simulink model "VCU_limit_torque"  (R2020a)
settings: Solver=FixedStepDiscrete  StartTime=0.0  StopTime=Parm_cnv_simulink_stopTime  FixedStep=Const_cnv_fundmt_stepSize  RelTol=1e-3  EnableMultiTasking=on
InitFcn:
  | preLoadFun
undefined symbols (not defined in the file or in its folder): IO397
libraries: speedgoatlib_IO691 x8, canmsglib x8, speedgoatlib_fpga x1
Description:
  | - Add preLoadFun.m into Callbacks InitFcn
  | - Combine Sensata and Pirelle sensor inputs into one subsystem
  | - Two enumerators: defEnum_fun_tbm.m && def_vehFun_Enum.m
settings Model: SimulationMode=external  PauseTimes=49.73  NumberOfSteps=20  EnablePacing=on  PacingRate=112  Creator=jianjun.gao  LastModifiedBy=bowen.zheng
settings SolverCC: ConcurrentTasks=on  AlgebraicLoopSolver=LineSearch  AutoInsertRateTranBlk=on
settings DataIOCC: LimitDataPoints=on  SaveFormat=StructureWithTime  ReturnWorkspaceOutputs=off
settings OptimizationCC: BlockReduction=off  DefaultUnderspecifiedDataType=single  OptimizeBlockIOStorage=off  EnhancedBackFolding=on  PassReuseOutputArgsThreshold=0  ExpressionDepthLimit=2147483647  OptimizeBlockOrder=speed  DifferentSizesBufferReuse=on
settings DebuggingCC: UnderspecifiedInitializationDetection=Classic  MergeDetectMultiDrivingBlocksExec=none  SolverPrmCheckMsg=warning  ParameterTunabilityLossMsg=error  FcnCallInpInsideContextMsg=warning  BusObjectLabelMismatch=error  AllowSymbolicDim=off  StateNameClashWarn=warning  SFUnexpectedBacktrackingDiag=warning  SFNoUnconditionalDefaultTransitionDiag=warning  SFExecutionAtInitializationDiag=none  ArithmeticOperatorsInVariantConditions=warning
settings HardwareCC: ProdBitPerPointer=32  ProdBitPerSizeT=32  ProdBitPerPtrDiffT=32  ProdLargestAtomicFloat=None  ProdWordSize=32  ProdLongLongMode=on  ProdHWDeviceType=Generic->32-bit x86 compatible
settings ModelReferenceCC: PropagateSignalLabelsOutOfModel=off
settings SFSimCC: SimUseLocalCustomCode=off  MATLABDynamicMemAlloc=off  CustomCodeUndefinedFunction=UseInterfaceOnly
settings RTWCC: Description=Simulink Real-Time  SystemTargetFile=slrt.tlc  PackageName=addn_compled  TemplateMakefile=slrt_default_tmf  RTWUseLocalCustomCode=off  RTWUseSimCustomCode=on  BuildConfiguration=Faster Runs  CodeExecutionProfiling=on  RTWCompilerOptimization=on
settings CodeAppCC: ForceParamTrailComments=on  MaxIdLength=63  OperatorAnnotations=on
settings SimulinkRealTimeCC: SupportVariableSizeSignals=on  RL32LogTETModifier=off  xPCConcurrentTasks=on
settings ConfigComp: CovMetricSettings=dw  CovHtmlReporting=on  CovSaveCumulativeToWorkspaceVar=on  CovSaveSingleToWorkspaceVar=on  CovExternalEMLEnable=off
settings SimscapeCC: SimscapeNormalizeSystem=off
settings ConfigurationSet: Description=SimMechanics 2G

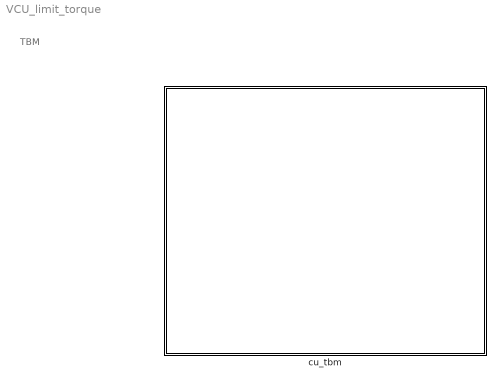
== system VCU_limit_torque ==
  note: TBM
  cu_tbm : Subsystem

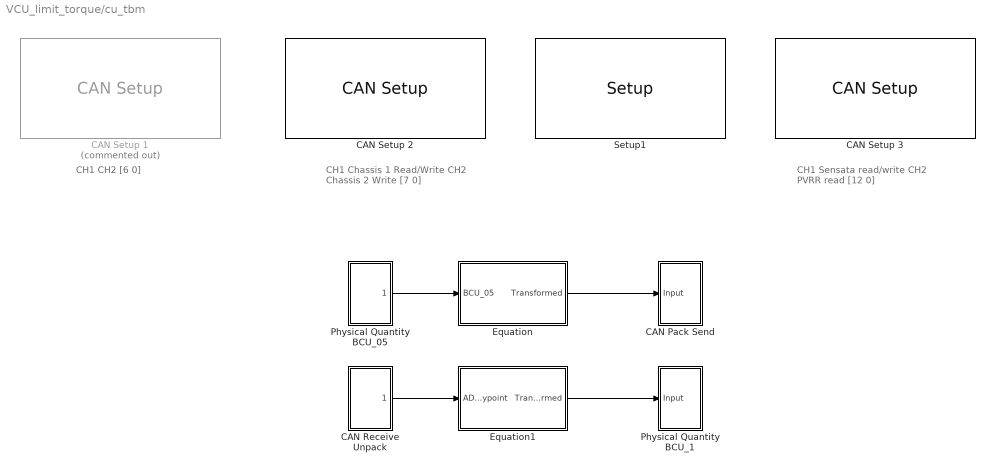
== system VCU_limit_torque/cu_tbm ==
  note: CH1
      | CH2
      | [6 0]
  note: CH1 Chassis 1 Read/Write
      | CH2 Chassis 2 Write
      | [7 0]
  note: CH1 Sensata read/write
      | CH2  PVRR read
      | [12 0]
  CAN Pack Send : Subsystem
  CAN Receive Unpack : Subsystem
  CAN Setup 1 : speedgoatlib_IO691/CAN Setup   Commented=on  moduletype=IO691  id=1  pciSlot=[6 0]  chn1=CAN (HS)  chn2=CAN (HS)  chn3=Disabled  chn4=Disabled  initStruct=[]  termStruct=[]  ArbitrationbdrChn1=500 kBaud  ArbitrationManbdrChn1=[2,16,63,16]  FdbdrChn1=5.0 MBaud  FdManbdrChn1=[2,2,5,2]  ArbitrationbdrChn2=500 kBaud  ArbitrationManbdrChn2=[2,16,63,16]  FdbdrChn2=5.0 MBaud  FdManbdrChn2=[2,2,5,2]  ArbitrationbdrChn3=1.0 MBaud  ArbitrationManbdrChn3=[2,8,31,8]  FdbdrChn3=5.0 MBaud  FdManbdrChn3=[2,2,5,2]  ArbitrationbdrChn4=1.0 MBaud  ArbitrationManbdrChn4=[2,8,31,8]  FdbdrChn4=5.0 MBaud  FdManbdrChn4=[2,2,5,2]  moduleInitValues=[691 1 6 0]
      settings: SourceProductName=Simulink Real-Time: Speedgoat I/O Blockset
  CAN Setup 2 : speedgoatlib_IO691/CAN Setup   moduletype=IO691  id=2  pciSlot=[7 0]  chn1=CAN (HS)  chn2=CAN (HS)  chn3=Disabled  chn4=Disabled  initStruct=[]  termStruct=[]  ArbitrationbdrChn1=500 kBaud  ArbitrationManbdrChn1=[2,16,63,16]  FdbdrChn1=5.0 MBaud  FdManbdrChn1=[2,2,5,2]  ArbitrationbdrChn2=500 kBaud  ArbitrationManbdrChn2=[2,16,63,16]  FdbdrChn2=5.0 MBaud  FdManbdrChn2=[2,2,5,2]  ArbitrationbdrChn3=1.0 MBaud  ArbitrationManbdrChn3=[2,8,31,8]  FdbdrChn3=5.0 MBaud  FdManbdrChn3=[2,2,5,2]  ArbitrationbdrChn4=1.0 MBaud  ArbitrationManbdrChn4=[2,8,31,8]  FdbdrChn4=5.0 MBaud  FdManbdrChn4=[2,2,5,2]  moduleInitValues=[691 2 7 0]
      settings: SourceProductName=Simulink Real-Time: Speedgoat I/O Blockset
  CAN Setup 3 : speedgoatlib_IO691/CAN Setup   moduletype=IO691  id=4  pciSlot=[12 0]  chn1=CAN (HS)  chn2=CAN (HS)  chn3=Disabled  chn4=Disabled  initStruct=[]  termStruct=[]  ArbitrationbdrChn1=500 kBaud  ArbitrationManbdrChn1=[2,16,63,16]  FdbdrChn1=5.0 MBaud  FdManbdrChn1=[2,2,5,2]  ArbitrationbdrChn2=1.0 MBaud  ArbitrationManbdrChn2=[2,8,31,8]  FdbdrChn2=5.0 MBaud  FdManbdrChn2=[2,2,5,2]  ArbitrationbdrChn3=1.0 MBaud  ArbitrationManbdrChn3=[2,8,31,8]  FdbdrChn3=5.0 MBaud  FdManbdrChn3=[2,2,5,2]  ArbitrationbdrChn4=1.0 MBaud  ArbitrationManbdrChn4=[2,8,31,8]  FdbdrChn4=5.0 MBaud  FdManbdrChn4=[2,2,5,2]  moduleInitValues=[691 4 12 0]
      settings: SourceProductName=Simulink Real-Time: Speedgoat I/O Blockset
  Equation : Subsystem
  Equation1 : Subsystem
  Physical Quantity BCU_05 : Subsystem
  Physical Quantity BCU_1 : Subsystem
  Setup1 : speedgoatlib_fpga/Setup/Setup  board=IO397-50k  id=3  device_id=1  frontIO=None  rearIO=None  bitstreamFile=speedgoat_IO397_50k_all_io.mat  rev=2.1  timestamp_string=06/12/19 11:07:30  fpgaFreq=75 MHz  fpgaTick=13.33 ns  ProgSpiFlash=off  ProgBPIFlash=off  pciSlot=-1  PullRPort0=pull-up 3.3V  VioPort0=3.3V  PullRPort1=pull-up 3.3V  VioPort1=3.3V  PullRPort2=pull-up 3.3V  VioPort2=3.3V  PullRPort3=pull-up 3.3V  VioPort3=3.3V  PullRPort4=pull-up 3.3V  VioPort4=3.3V  PullRPort5=pull-up 3.3V  VioPort5=3.3V  PullRPort6=pull-up 3.3V  VioPort6=3.3V  PullRPort15=pull-up 3.3V  PullRPort31=pull-up 3.3V  PullRPort47=pull-up 3.3V  PullRPort63=pull-up 3.3V
      settings: SourceProductName=Simulink Real-Time: Speedgoat Library
  wires:
  Physical Quantity BCU_05/1(BCU_05) -> Equation/1(BCU_05)
  Equation/1(Transformed) -> CAN Pack Send/1(Input)
  CAN Receive Unpack/1(Output) -> Equation1/1(ADC_Waypoint)
  Equation1/1(Transformed) -> Physical Quantity BCU_1/1(Input)

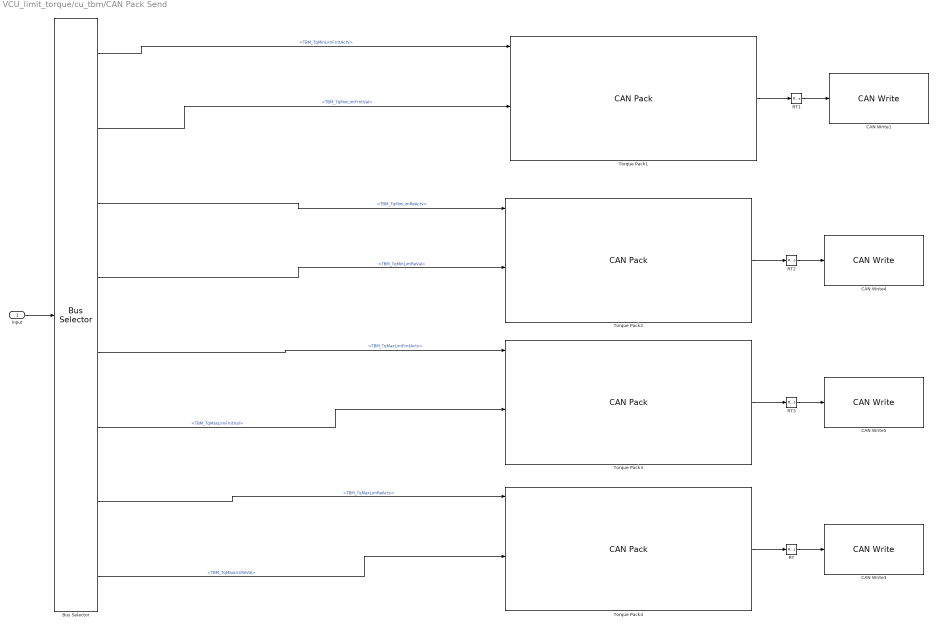
== system VCU_limit_torque/cu_tbm/CAN Pack Send ==
  Input : Inport
  Bus Selector : BusSelector  OutputSignals=TBM_TqMinLimFrntActv,TBM_TqMinLimFrntVal,TBM_TqMinLimReActv,TBM_TqMinLimReVal,TBM_TqMaxLimFrntActv,TBM_TqMaxLimFrntVal,TBM_TqMaxLimReActv,TBM_TqMaxLimReVal
  CAN Write{1,3..5} (4 alike) : speedgoatlib_IO691/CAN Write  id=2  ts=0.02  channel=1  messageType=CAN  enableStatusPort=off  canType=CAN (HS)  initValues=[691 2 0.02 0 1 1 0]
      settings: SourceProductName=Simulink Real-Time: Speedgoat I/O Blockset
  RT{,1..3} (4 alike) : RateTransition  OutPortSampleTime=0.02
  Torque Pack1 : canmsglib/CAN Pack  CANdbFile=.\support\dbc\NIO_NT2_Chassis2_CAN_Official_Release_V_1_1_DA_02.dbc  MsgList=ADC1_WayPoint01  MsgName=ADC1_WayPoint01  MsgIDType=Standard (11-bit identifier)  MsgIdentifier=214  MsgLength=8  Remote=off  ApplyMinMax=off  BusOutput=off  SignalInfo={'LD_Confidence_1','24','4','BE','unsigned','Standard','0','0.1','0','0','1.5';'LD_First_End_1','51','7','BE','unsigned','Standard','0','1','0','0','127';'LD_First_Start_1','16','8','BE','unsigned','Standard','0','0.1','0','0','25.5';'LD_First_Type_1','28','4','BE','unsigned','Standard','0','1','0','0','15';'LD_Line_First_C0_1','56','11','BE','unsigned','Standard','0','0.01','-10.24','-10.24','10.23';'LD_Line_First_C1_1','43','13','BE','unsigned','Standard','0','0.0001','-0.4096','-0.4096','0.4095';'LD_Line_First_C2_1','0','8','BE','unsigned','Standard','0','0.0001','-0.0128','-0.0128','0.0127';'LD_Line_First_C3_1','8','8','BE','unsigned','Standard','0','1e-06','-0.000128','-0.000128','0.000127'}
      settings: SourceProductBaseCode=ME,VN  DataFormat=CANdb specified signals
  Torque Pack2 : canmsglib/CAN Pack  CANdbFile=.\support\dbc\NIO_NT2_Chassis2_CAN_Official_Release_V_1_1_DA_02.dbc  MsgList=ADC1_WayPoint02  MsgName=ADC1_WayPoint02  MsgIDType=Standard (11-bit identifier)  MsgIdentifier=215  MsgLength=8  Remote=off  ApplyMinMax=off  BusOutput=off  SignalInfo={'LD_Confidence_2','24','4','BE','unsigned','Standard','0','0.1','0','0','1.5';'LD_First_End_2','51','7','BE','unsigned','Standard','0','1','0','0','127';'LD_First_Start_2','16','8','BE','unsigned','Standard','0','0.1','0','0','25.5';'LD_First_Type_2','28','4','BE','unsigned','Standard','0','1','0','0','15';'LD_Line_First_C0_2','56','11','BE','unsigned','Standard','0','0.01','-10.24','-10.24','10.23';'LD_Line_First_C1_2','43','13','BE','unsigned','Standard','0','0.0001','-0.4096','-0.4096','0.4095';'LD_Line_First_C2_2','0','8','BE','unsigned','Standard','0','0.0001','-0.0128','-0.0128','0.0127';'LD_Line_First_C3_2','8','8','BE','unsigned','Standard','0','1e-06','-0.000128','-0.000128','0.000127'}
      settings: SourceProductBaseCode=ME,VN  DataFormat=CANdb specified signals
  Torque Pack3 : canmsglib/CAN Pack  CANdbFile=.\support\dbc\NIO_NT2_Chassis2_CAN_Official_Release_V_1_1_DA_02.dbc  MsgList=ADC1_WayPoint03  MsgName=ADC1_WayPoint03  MsgIDType=Standard (11-bit identifier)  MsgIdentifier=216  MsgLength=8  Remote=off  ApplyMinMax=off  BusOutput=off  SignalInfo={'LD_Confidence_3','24','4','BE','unsigned','Standard','0','0.1','0','0','1.5';'LD_First_End_3','51','7','BE','unsigned','Standard','0','1','0','0','127';'LD_First_Start_3','16','8','BE','unsigned','Standard','0','0.1','0','0','25.5';'LD_First_Type_3','28','4','BE','unsigned','Standard','0','1','0','0','15';'LD_Line_First_C0_3','56','11','BE','unsigned','Standard','0','0.01','-10.24','-10.24','10.23';'LD_Line_First_C1_3','43','13','BE','unsigned','Standard','0','0.0001','-0.4096','-0.4096','0.4095';'LD_Line_First_C2_3','0','8','BE','unsigned','Standard','0','0.0001','-0.0128','-0.0128','0.0127';'LD_Line_First_C3_3','8','8','BE','unsigned','Standard','0','1e-06','-0.000128','-0.000128','0.000127'}
      settings: SourceProductBaseCode=ME,VN  DataFormat=CANdb specified signals
  Torque Pack4 : canmsglib/CAN Pack  CANdbFile=.\support\dbc\NIO_NT2_Chassis2_CAN_Official_Release_V_1_1_DA_02.dbc  MsgList=ADC1_WayPoint04  MsgName=ADC1_WayPoint04  MsgIDType=Standard (11-bit identifier)  MsgIdentifier=217  MsgLength=8  Remote=off  ApplyMinMax=off  BusOutput=off  SignalInfo={'LD_Confidence_4','24','4','BE','unsigned','Standard','0','0.1','0','0','1.5';'LD_First_End_4','51','7','BE','unsigned','Standard','0','1','0','0','127';'LD_First_Start_4','16','8','BE','unsigned','Standard','0','0.1','0','0','25.5';'LD_First_Type_4','28','4','BE','unsigned','Standard','0','1','0','0','15';'LD_Line_First_C0_4','56','11','BE','unsigned','Standard','0','0.01','-10.24','-10.24','10.23';'LD_Line_First_C1_4','43','13','BE','unsigned','Standard','0','0.0001','-0.4096','-0.4096','0.4095';'LD_Line_First_C2_4','0','8','BE','unsigned','Standard','0','0.0001','-0.0128','-0.0128','0.0127';'LD_Line_First_C3_4','8','8','BE','unsigned','Standard','0','1e-06','-0.000128','-0.000128','0.000127'}
      settings: SourceProductBaseCode=ME,VN  DataFormat=CANdb specified signals
  wires:
  RT/1 -> CAN Write3/1
  RT3/1 -> CAN Write5/1
  Torque Pack3/1 -> RT3/1
  Torque Pack4/1 -> RT/1
  Torque Pack2/1 -> RT2/1
  RT2/1 -> CAN Write4/1
  Input/1 -> Bus Selector/1
  Bus Selector/1 -> Torque Pack1/1  "<TBM_TqMinLimFrntActv>"
  RT1/1 -> CAN Write1/1
  Torque Pack1/1 -> RT1/1
  Bus Selector/2 -> Torque Pack1/5  "<TBM_TqMinLimFrntVal>"
  Bus Selector/3 -> Torque Pack2/1  "<TBM_TqMinLimReActv>"
  Bus Selector/4 -> Torque Pack2/5  "<TBM_TqMinLimReVal>"
  Bus Selector/5 -> Torque Pack3/1  "<TBM_TqMaxLimFrntActv>"
  Bus Selector/6 -> Torque Pack3/5  "<TBM_TqMaxLimFrntVal>"
  Bus Selector/7 -> Torque Pack4/1  "<TBM_TqMaxLimReActv>"
  Bus Selector/8 -> Torque Pack4/5  "<TBM_TqMaxLimReVal>"

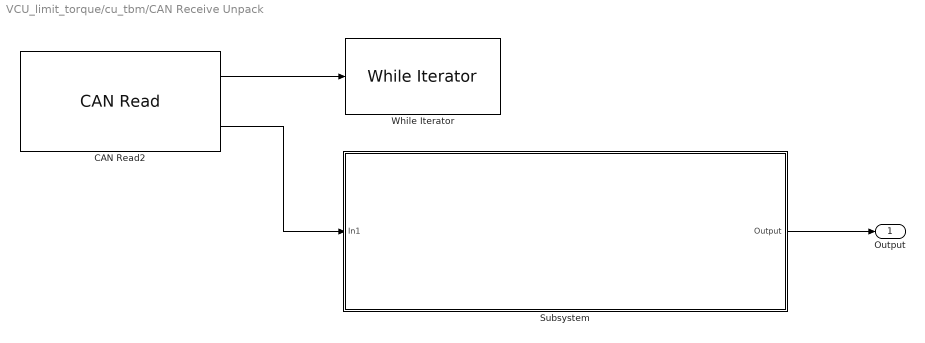
== system VCU_limit_torque/cu_tbm/CAN Receive Unpack ==
  CAN Read2 : speedgoatlib_IO691/CAN Read  id=2  ts=-1  channel=1  messageType=CAN  canType=CAN (HS)  initValues=[691 2 -1 0 1 1]
      settings: SourceProductName=Simulink Real-Time: Speedgoat I/O Blockset
  Subsystem : Subsystem
  While Iterator : WhileIterator  MaxIters=-1  WhileBlockType=do-while
  Output : Outport
  wires:
  CAN Read2/2 -> Subsystem/1(In1)
  CAN Read2/1 -> While Iterator/1
  Subsystem/1(Output) -> Output/1

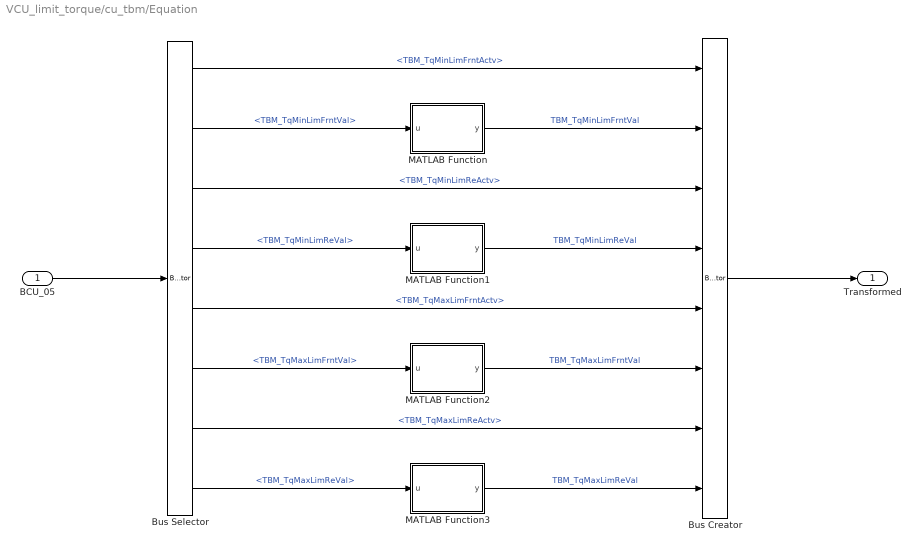
== system VCU_limit_torque/cu_tbm/Equation ==
  BCU_05 : Inport
  Bus Creator : BusCreator  Inputs=8
  Bus Selector : BusSelector  OutputSignals=TBM_TqMinLimFrntActv,TBM_TqMinLimFrntVal,TBM_TqMinLimReActv,TBM_TqMinLimReVal,TBM_TqMaxLimFrntActv,TBM_TqMaxLimFrntVal,TBM_TqMaxLimReActv,TBM_TqMaxLimReVal
  MATLAB Function : MATLAB Function  TreatAsAtomicUnit=on
  MATLAB Function1 : MATLAB Function  TreatAsAtomicUnit=on
  MATLAB Function2 : MATLAB Function  TreatAsAtomicUnit=on
  MATLAB Function3 : MATLAB Function  TreatAsAtomicUnit=on
  Transformed : Outport
  wires:
  BCU_05/1 -> Bus Selector/1
  Bus Creator/1 -> Transformed/1
  Bus Selector/1 -> Bus Creator/1  "<TBM_TqMinLimFrntActv>"
  Bus Selector/3 -> Bus Creator/3  "<TBM_TqMinLimReActv>"
  Bus Selector/5 -> Bus Creator/5  "<TBM_TqMaxLimFrntActv>"
  Bus Selector/7 -> Bus Creator/7  "<TBM_TqMaxLimReActv>"
  Bus Selector/2 -> MATLAB Function/1(u)  "<TBM_TqMinLimFrntVal>"
  MATLAB Function/1(y) -> Bus Creator/2  "TBM_TqMinLimFrntVal"
  Bus Selector/8 -> MATLAB Function3/1(u)  "<TBM_TqMaxLimReVal>"
  Bus Selector/6 -> MATLAB Function2/1(u)  "<TBM_TqMaxLimFrntVal>"
  Bus Selector/4 -> MATLAB Function1/1(u)  "<TBM_TqMinLimReVal>"
  MATLAB Function1/1(y) -> Bus Creator/4  "TBM_TqMinLimReVal"
  MATLAB Function2/1(y) -> Bus Creator/6  "TBM_TqMaxLimFrntVal"
  MATLAB Function3/1(y) -> Bus Creator/8  "TBM_TqMaxLimReVal"

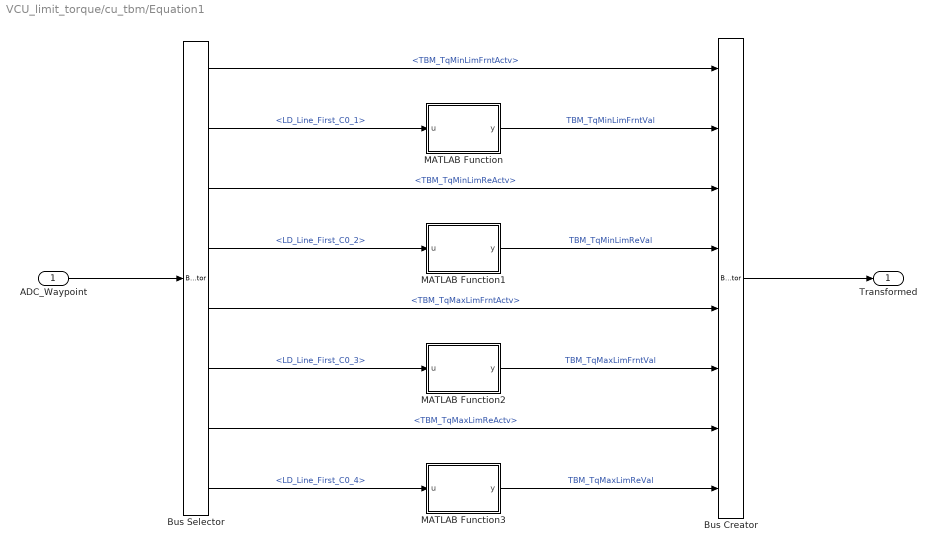
== system VCU_limit_torque/cu_tbm/Equation1 ==
  ADC_Waypoint : Inport
  Bus Creator : BusCreator  Inputs=8
  Bus Selector : BusSelector  OutputSignals=TBM_TqMinLimFrntActv,LD_Line_First_C0_1,TBM_TqMinLimReActv,LD_Line_First_C0_2,TBM_TqMaxLimFrntActv,LD_Line_First_C0_3,TBM_TqMaxLimReActv,LD_Line_First_C0_4
  MATLAB Function : MATLAB Function  TreatAsAtomicUnit=on
  MATLAB Function1 : MATLAB Function  TreatAsAtomicUnit=on
  MATLAB Function2 : MATLAB Function  TreatAsAtomicUnit=on
  MATLAB Function3 : MATLAB Function  TreatAsAtomicUnit=on
  Transformed : Outport
  wires:
  ADC_Waypoint/1 -> Bus Selector/1
  Bus Creator/1 -> Transformed/1
  Bus Selector/1 -> Bus Creator/1  "<TBM_TqMinLimFrntActv>"
  Bus Selector/3 -> Bus Creator/3  "<TBM_TqMinLimReActv>"
  Bus Selector/5 -> Bus Creator/5  "<TBM_TqMaxLimFrntActv>"
  Bus Selector/7 -> Bus Creator/7  "<TBM_TqMaxLimReActv>"
  Bus Selector/2 -> MATLAB Function/1(u)  "<LD_Line_First_C0_1>"
  MATLAB Function/1(y) -> Bus Creator/2  "TBM_TqMinLimFrntVal"
  Bus Selector/8 -> MATLAB Function3/1(u)  "<LD_Line_First_C0_4>"
  Bus Selector/6 -> MATLAB Function2/1(u)  "<LD_Line_First_C0_3>"
  Bus Selector/4 -> MATLAB Function1/1(u)  "<LD_Line_First_C0_2>"
  MATLAB Function1/1(y) -> Bus Creator/4  "TBM_TqMinLimReVal"
  MATLAB Function2/1(y) -> Bus Creator/6  "TBM_TqMaxLimFrntVal"
  MATLAB Function3/1(y) -> Bus Creator/8  "TBM_TqMaxLimReVal"

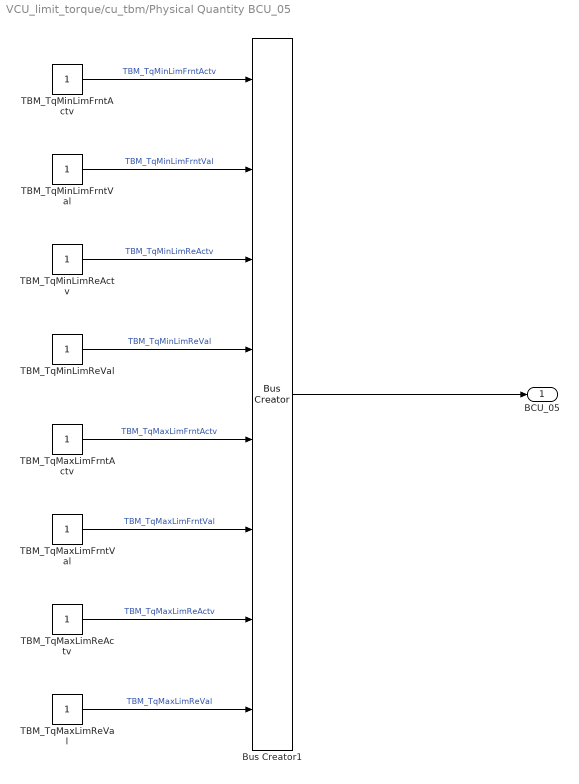
== system VCU_limit_torque/cu_tbm/Physical Quantity BCU_05 ==
  Bus Creator1 : BusCreator  Inputs=8
  TBM_TqMaxLimFrntActv : Constant  OutDataTypeStr=single
  TBM_TqMaxLimFrntVal : Constant  OutDataTypeStr=single
  TBM_TqMaxLimReActv : Constant  OutDataTypeStr=single
  TBM_TqMaxLimReVal : Constant  OutDataTypeStr=single
  TBM_TqMinLimFrntActv : Constant  OutDataTypeStr=single
  TBM_TqMinLimFrntVal : Constant  OutDataTypeStr=single
  TBM_TqMinLimReActv : Constant  OutDataTypeStr=single
  TBM_TqMinLimReVal : Constant  OutDataTypeStr=single
  BCU_05 : Outport  OutDataTypeStr=single  PortDimensions=8
  wires:
  TBM_TqMaxLimReVal/1 -> Bus Creator1/8  "TBM_TqMaxLimReVal"
  Bus Creator1/1 -> BCU_05/1
  TBM_TqMinLimFrntVal/1 -> Bus Creator1/2  "TBM_TqMinLimFrntVal"
  TBM_TqMinLimReVal/1 -> Bus Creator1/4  "TBM_TqMinLimReVal"
  TBM_TqMinLimReActv/1 -> Bus Creator1/3  "TBM_TqMinLimReActv"
  TBM_TqMaxLimFrntActv/1 -> Bus Creator1/5  "TBM_TqMaxLimFrntActv"
  TBM_TqMaxLimReActv/1 -> Bus Creator1/7  "TBM_TqMaxLimReActv"
  TBM_TqMinLimFrntActv/1 -> Bus Creator1/1  "TBM_TqMinLimFrntActv"
  TBM_TqMaxLimFrntVal/1 -> Bus Creator1/6  "TBM_TqMaxLimFrntVal"

== system VCU_limit_torque/cu_tbm/Physical Quantity BCU_1 ==
  Input : Inport
  Bus Selector : BusSelector  OutputSignals=TBM_TqMinLimFrntActv,TBM_TqMinLimFrntVal,TBM_TqMinLimReActv,TBM_TqMinLimReVal,TBM_TqMaxLimFrntActv,TBM_TqMaxLimFrntVal,TBM_TqMaxLimReActv,TBM_TqMaxLimReVal
  wires:
  Bus Selector/8 -> ?  "<TBM_TqMaxLimReVal>"
  Bus Selector/2 -> ?  "<TBM_TqMinLimFrntVal>"
  Bus Selector/4 -> ?  "<TBM_TqMinLimReVal>"
  Bus Selector/3 -> ?  "<TBM_TqMinLimReActv>"
  Bus Selector/5 -> ?  "<TBM_TqMaxLimFrntActv>"
  Bus Selector/7 -> ?  "<TBM_TqMaxLimReActv>"
  Bus Selector/1 -> ?  "<TBM_TqMinLimFrntActv>"
  Bus Selector/6 -> ?  "<TBM_TqMaxLimFrntVal>"
  Input/1 -> Bus Selector/1

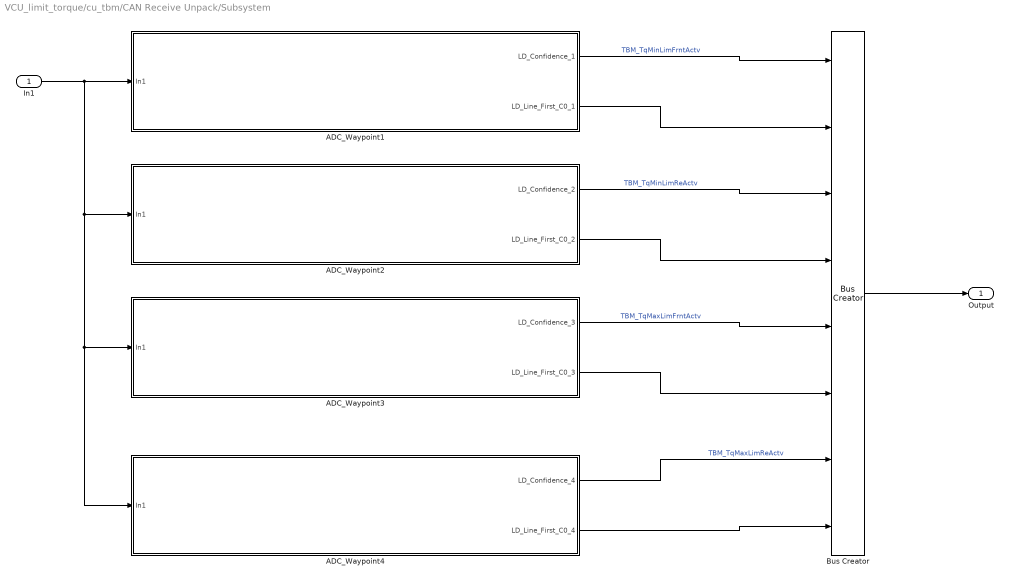
== system VCU_limit_torque/cu_tbm/CAN Receive Unpack/Subsystem ==
  In1 : Inport
  ADC_Waypoint1 : Subsystem
  ADC_Waypoint2 : Subsystem
  ADC_Waypoint3 : Subsystem
  ADC_Waypoint4 : Subsystem
  Bus Creator : BusCreator  Inputs=8
  Output : Outport
  wires:
  In1/1 -> ADC_Waypoint4/1(In1), ADC_Waypoint3/1(In1), ADC_Waypoint2/1(In1), ADC_Waypoint1/1(In1)
  ADC_Waypoint1/1(LD_Confidence_1) -> Bus Creator/1  "TBM_TqMinLimFrntActv"
  ADC_Waypoint1/2(LD_Line_First_C0_1) -> Bus Creator/2
  ADC_Waypoint2/1(LD_Confidence_2) -> Bus Creator/3  "TBM_TqMinLimReActv"
  ADC_Waypoint2/2(LD_Line_First_C0_2) -> Bus Creator/4
  ADC_Waypoint3/1(LD_Confidence_3) -> Bus Creator/5  "TBM_TqMaxLimFrntActv"
  ADC_Waypoint3/2(LD_Line_First_C0_3) -> Bus Creator/6
  ADC_Waypoint4/1(LD_Confidence_4) -> Bus Creator/7  "TBM_TqMaxLimReActv"
  ADC_Waypoint4/2(LD_Line_First_C0_4) -> Bus Creator/8
  Bus Creator/1 -> Output/1

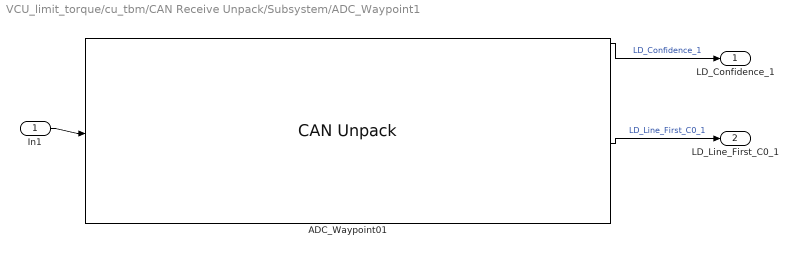
== system VCU_limit_torque/cu_tbm/CAN Receive Unpack/Subsystem/ADC_Waypoint1 ==
  In1 : Inport
  ADC_Waypoint01 : canmsglib/CAN Unpack  CANdbFile=C:\Users\bowen.zheng\Desktop\spdGoat_prj_20230605\spdGoat_prj_20230605\support\dbc\NIO_NT2_Chassis2_CAN_Official_Release_V_1_1_DA_02.dbc  MsgList=ADC1_WayPoint01  MsgName=ADC1_WayPoint01  MsgIDType=Standard (11-bit identifier)  MsgIdentifier=214  MsgLength=8  SignalInfo={'LD_Confidence_1','24','4','BE','unsigned','Standard','0','0.1','0','0','1.5';'LD_First_End_1','51','7','BE','unsigned','Standard','0','1','0','0','127';'LD_First_Start_1','16','8','BE','unsigned','Standard','0','0.1','0','0','25.5';'LD_First_Type_1','28','4','BE','unsigned','Standard','0','1','0','0','15';'LD_Line_First_C0_1','56','11','BE','unsigned','Standard','0','0.01','-10.24','-10.24','10.23';'LD_Line_First_C1_1','43','13','BE','unsigned','Standard','0','0.0001','-0.4096','-0.4096','0.4095';'LD_Line_First_C2_1','0','8','BE','unsigned','Standard','0','0.0001','-0.0128','-0.0128','0.0127';'LD_Line_First_C3_1','8','8','BE','unsigned','Standard','0','1e-06','-0.000128','-0.000128','0.000127'}  IDPort=off  TimestampPort=off  ErrorPort=off  RemotePort=off  LengthPort=off  StatusPort=off  ApplyMinMax=off
      settings: SourceProductBaseCode=ME,VN  DataFormat=CANdb specified signals
  LD_Confidence_1 : Outport
  LD_Line_First_C0_1 : Outport  Port=2
  wires:
  In1/1 -> ADC_Waypoint01/1
  ADC_Waypoint01/1 -> LD_Confidence_1/1  "LD_Confidence_1"
  ADC_Waypoint01/5 -> LD_Line_First_C0_1/1  "LD_Line_First_C0_1"

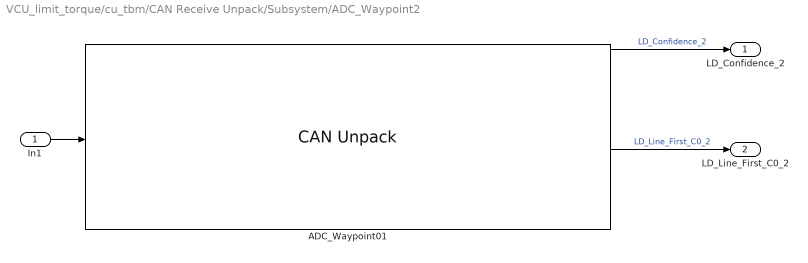
== system VCU_limit_torque/cu_tbm/CAN Receive Unpack/Subsystem/ADC_Waypoint2 ==
  In1 : Inport
  ADC_Waypoint01 : canmsglib/CAN Unpack  CANdbFile=C:\Users\bowen.zheng\Desktop\spdGoat_prj_20230605\spdGoat_prj_20230605\support\dbc\NIO_NT2_Chassis2_CAN_Official_Release_V_1_1_DA_02.dbc  MsgList=ADC1_WayPoint02  MsgName=ADC1_WayPoint02  MsgIDType=Standard (11-bit identifier)  MsgIdentifier=215  MsgLength=8  SignalInfo={'LD_Confidence_2','24','4','BE','unsigned','Standard','0','0.1','0','0','1.5';'LD_First_End_2','51','7','BE','unsigned','Standard','0','1','0','0','127';'LD_First_Start_2','16','8','BE','unsigned','Standard','0','0.1','0','0','25.5';'LD_First_Type_2','28','4','BE','unsigned','Standard','0','1','0','0','15';'LD_Line_First_C0_2','56','11','BE','unsigned','Standard','0','0.01','-10.24','-10.24','10.23';'LD_Line_First_C1_2','43','13','BE','unsigned','Standard','0','0.0001','-0.4096','-0.4096','0.4095';'LD_Line_First_C2_2','0','8','BE','unsigned','Standard','0','0.0001','-0.0128','-0.0128','0.0127';'LD_Line_First_C3_2','8','8','BE','unsigned','Standard','0','1e-06','-0.000128','-0.000128','0.000127'}  IDPort=off  TimestampPort=off  ErrorPort=off  RemotePort=off  LengthPort=off  StatusPort=off  ApplyMinMax=off
      settings: SourceProductBaseCode=ME,VN  DataFormat=CANdb specified signals
  LD_Confidence_2 : Outport
  LD_Line_First_C0_2 : Outport  Port=2
  wires:
  In1/1 -> ADC_Waypoint01/1
  ADC_Waypoint01/1 -> LD_Confidence_2/1  "LD_Confidence_2"
  ADC_Waypoint01/5 -> LD_Line_First_C0_2/1  "LD_Line_First_C0_2"

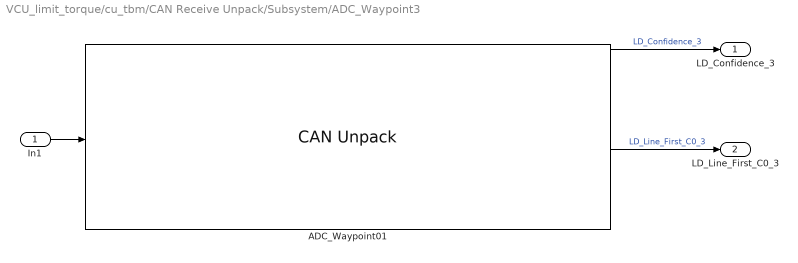
== system VCU_limit_torque/cu_tbm/CAN Receive Unpack/Subsystem/ADC_Waypoint3 ==
  In1 : Inport
  ADC_Waypoint01 : canmsglib/CAN Unpack  CANdbFile=C:\Users\bowen.zheng\Desktop\spdGoat_prj_20230605\spdGoat_prj_20230605\support\dbc\NIO_NT2_Chassis2_CAN_Official_Release_V_1_1_DA_02.dbc  MsgList=ADC1_WayPoint03  MsgName=ADC1_WayPoint03  MsgIDType=Standard (11-bit identifier)  MsgIdentifier=216  MsgLength=8  SignalInfo={'LD_Confidence_3','24','4','BE','unsigned','Standard','0','0.1','0','0','1.5';'LD_First_End_3','51','7','BE','unsigned','Standard','0','1','0','0','127';'LD_First_Start_3','16','8','BE','unsigned','Standard','0','0.1','0','0','25.5';'LD_First_Type_3','28','4','BE','unsigned','Standard','0','1','0','0','15';'LD_Line_First_C0_3','56','11','BE','unsigned','Standard','0','0.01','-10.24','-10.24','10.23';'LD_Line_First_C1_3','43','13','BE','unsigned','Standard','0','0.0001','-0.4096','-0.4096','0.4095';'LD_Line_First_C2_3','0','8','BE','unsigned','Standard','0','0.0001','-0.0128','-0.0128','0.0127';'LD_Line_First_C3_3','8','8','BE','unsigned','Standard','0','1e-06','-0.000128','-0.000128','0.000127'}  IDPort=off  TimestampPort=off  ErrorPort=off  RemotePort=off  LengthPort=off  StatusPort=off  ApplyMinMax=off
      settings: SourceProductBaseCode=ME,VN  DataFormat=CANdb specified signals
  LD_Confidence_3 : Outport
  LD_Line_First_C0_3 : Outport  Port=2
  wires:
  In1/1 -> ADC_Waypoint01/1
  ADC_Waypoint01/1 -> LD_Confidence_3/1  "LD_Confidence_3"
  ADC_Waypoint01/5 -> LD_Line_First_C0_3/1  "LD_Line_First_C0_3"

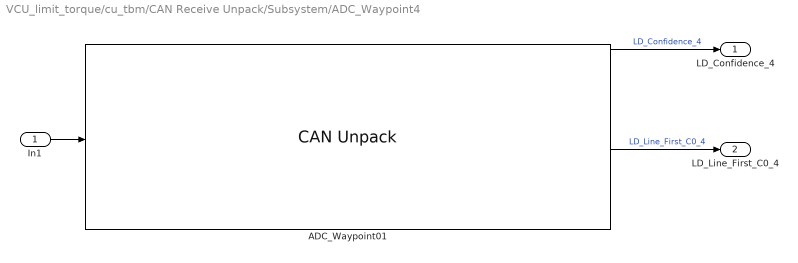
== system VCU_limit_torque/cu_tbm/CAN Receive Unpack/Subsystem/ADC_Waypoint4 ==
  In1 : Inport
  ADC_Waypoint01 : canmsglib/CAN Unpack  CANdbFile=C:\Users\bowen.zheng\Desktop\spdGoat_prj_20230605\spdGoat_prj_20230605\support\dbc\NIO_NT2_Chassis2_CAN_Official_Release_V_1_1_DA_02.dbc  MsgList=ADC1_WayPoint04  MsgName=ADC1_WayPoint04  MsgIDType=Standard (11-bit identifier)  MsgIdentifier=217  MsgLength=8  SignalInfo={'LD_Confidence_4','24','4','BE','unsigned','Standard','0','0.1','0','0','1.5';'LD_First_End_4','51','7','BE','unsigned','Standard','0','1','0','0','127';'LD_First_Start_4','16','8','BE','unsigned','Standard','0','0.1','0','0','25.5';'LD_First_Type_4','28','4','BE','unsigned','Standard','0','1','0','0','15';'LD_Line_First_C0_4','56','11','BE','unsigned','Standard','0','0.01','-10.24','-10.24','10.23';'LD_Line_First_C1_4','43','13','BE','unsigned','Standard','0','0.0001','-0.4096','-0.4096','0.4095';'LD_Line_First_C2_4','0','8','BE','unsigned','Standard','0','0.0001','-0.0128','-0.0128','0.0127';'LD_Line_First_C3_4','8','8','BE','unsigned','Standard','0','1e-06','-0.000128','-0.000128','0.000127'}  IDPort=off  TimestampPort=off  ErrorPort=off  RemotePort=off  LengthPort=off  StatusPort=off  ApplyMinMax=off
      settings: SourceProductBaseCode=ME,VN  DataFormat=CANdb specified signals
  LD_Confidence_4 : Outport
  LD_Line_First_C0_4 : Outport  Port=2
  wires:
  In1/1 -> ADC_Waypoint01/1
  ADC_Waypoint01/1 -> LD_Confidence_4/1  "LD_Confidence_4"
  ADC_Waypoint01/5 -> LD_Line_First_C0_4/1  "LD_Line_First_C0_4"

== matlab function VCU_limit_torque/cu_tbm/Equation/MATLAB Function1 ==
  data: u input; y output
function y = fcn(u)

 y = 0.01 * u - 6.04;

== matlab function VCU_limit_torque/cu_tbm/Equation/MATLAB Function2 ==
  data: u input; y output
function y = fcn(u)

 y = 0.01 * u - 6.04;

== matlab function VCU_limit_torque/cu_tbm/Equation/MATLAB Function3 ==
  data: u input; y output
function y = fcn(u)

 y = 0.01 * u - 6.04;

== matlab function VCU_limit_torque/cu_tbm/Equation1/MATLAB Function ==
  data: u input; y output
function y = fcn(u)

 y = (u + 6.04) / 0.01;

== matlab function VCU_limit_torque/cu_tbm/Equation1/MATLAB Function1 ==
  data: u input; y output
function y = fcn(u)

 y = (u + 6.04) / 0.01;

== matlab function VCU_limit_torque/cu_tbm/Equation1/MATLAB Function2 ==
  data: u input; y output
function y = fcn(u)

 y = (u + 6.04) / 0.01;

== matlab function VCU_limit_torque/cu_tbm/Equation1/MATLAB Function3 ==
  data: u input; y output
function y = fcn(u)

 y = (u + 6.04) / 0.01;

== matlab function VCU_limit_torque/cu_tbm/Equation/MATLAB Function ==
  data: u input; y output
function y = fcn(u)

 y = 0.01 * u - 6.04;
